simulink model "mpc_cvxgen"  (R2015b)
settings: Solver=VariableStepAuto  StartTime=0.0  StopTime=15  FixedStep=Ts  RelTol=1e-3
InitFcn:
  | mpc_trajectory_data_callback
values from neighbouring files (symbols this model uses):
  Ts = 0.1    [init_mpc_test.m]
undefined symbols (not defined in the file or in its folder): sCoeffs, sPolyorder, sTimes
undefined symbols (not defined in the file): CVXparameters
settings Model: Creator=Daniel  LastModifiedBy=mgreiff
settings SolverCC: AlgebraicLoopSolver=LineSearch

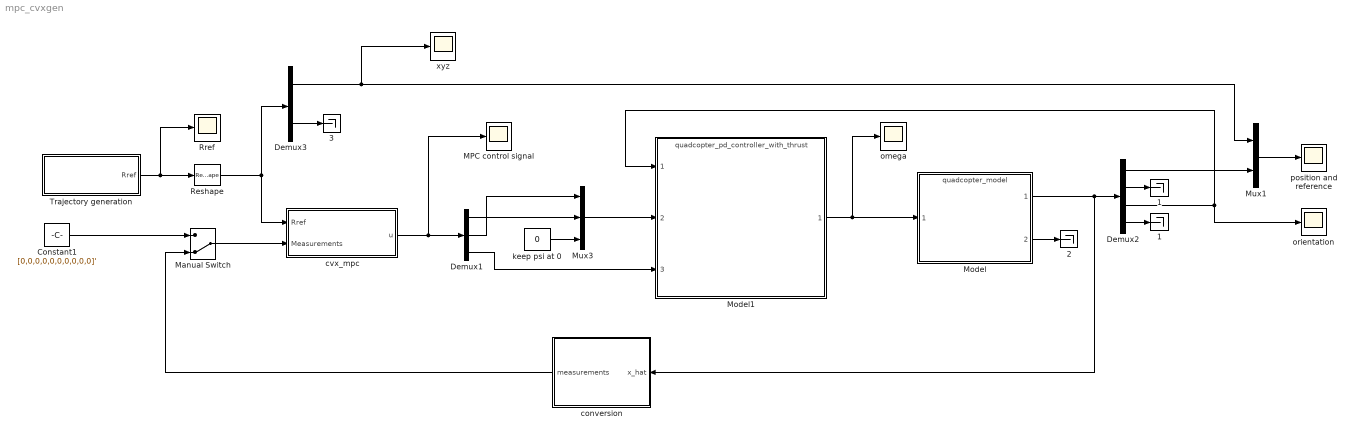
== system mpc_cvxgen ==
  "   1" : Terminator
  "   2" : Terminator
  "   3" : Terminator
  "  1" : Terminator
  Constant1 : Constant  Value=[0,0,0,0,0,0,0,0,0,0]'
  Demux1 : Demux  Outputs=3
  Demux2 : Demux  Outputs=[3,3,3,3]
  Demux3 : Demux  Outputs=[3,11*10-3]
  MPC control signal : Scope
  Manual Switch : ManualSwitch  CurrentSetting=0
  Model : ModelReference  ModelNameDialog=quadcopter_model.mdl  SimulationMode=Normal  ModelReferenceVersion=1.117  CopyOfModelName=quadcopter_model.mdl
  Model1 : ModelReference  ModelNameDialog=quadcopter_pd_controller_with_thrust.mdl  SimulationMode=Normal  ModelReferenceVersion=1.72  CopyOfModelName=quadcopter_pd_controller_with_thrust.mdl
  Mux1 : Mux  Inputs=2
  Mux3 : Mux  Inputs=3
  Reshape : Reshape
  Rref : Scope
  Trajectory generation : Subsystem
  conversion : Subsystem
  cvx_mpc : Subsystem  mask{md=CVXparameters}
      mask prompts: md "MPCData"
  keep psi at 0 : Constant  Value=0
  omega : Scope
  orientation : Scope
  position and reference : Scope
  xyz : Scope
  wires:
  Trajectory generation/1(Rref) -> Rref/1, Reshape/1
  cvx_mpc/1(u) -> MPC control signal/1, Demux1/1
  Demux1/3 -> Model1/3
  Mux3/1 -> Model1/2
  keep psi at 0/1 -> Mux3/3
  Demux1/2 -> Mux3/1
  Demux1/1 -> Mux3/2
  Demux2/2 -> "  1"/1
  Demux2/4 -> "   1"/1
  Demux2/3 -> Model1/1, orientation/1
  Model/1 -> Demux2/1, conversion/1(x_hat)
  Model/2 -> "   2"/1
  Model1/1 -> omega/1, Model/1
  Constant1/1 -> Manual Switch/1
  Manual Switch/1 -> cvx_mpc/2(Measurements)
  conversion/1(measurements) -> Manual Switch/2
  Reshape/1 -> Demux3/1, cvx_mpc/1(Rref)
  Demux3/2 -> "   3"/1
  Demux3/1 -> Mux1/1, xyz/1
  Demux2/1 -> Mux1/2
  Mux1/1 -> position and reference/1

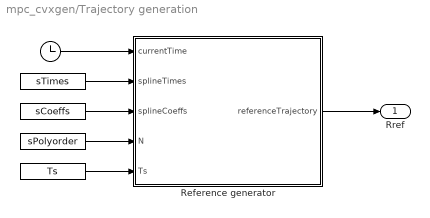
== system mpc_cvxgen/Trajectory generation ==
  " " : Constant  Value=Ts
  "  " : Constant  Value=sPolyorder
  "   " : Constant  Value=sCoeffs
  "    " : Constant  Value=sTimes
  "      " : Clock
  Reference generator : MATLAB Function  TreatAsAtomicUnit=on
  Rref : Outport
  wires:
  "      "/1 -> Reference generator/1(currentTime)
  "    "/1 -> Reference generator/2(splineTimes)
  "   "/1 -> Reference generator/3(splineCoeffs)
  "  "/1 -> Reference generator/4(N)
  " "/1 -> Reference generator/5(Ts)
  Reference generator/1(referenceTrajectory) -> Rref/1

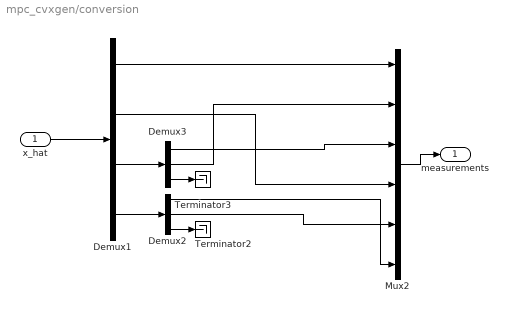
== system mpc_cvxgen/conversion ==
  x_hat : Inport
  Demux1 : Demux  Outputs=[3,3,3,3]
  Demux2 : Demux  Outputs=3
  Demux3 : Demux  Outputs=3
  Mux2 : Mux  Inputs=6
  Terminator2 : Terminator
  Terminator3 : Terminator
  measurements : Outport
  wires:
  Mux2/1 -> measurements/1
  x_hat/1 -> Demux1/1
  Demux1/1 -> Mux2/1
  Demux1/2 -> Mux2/4
  Demux2/3 -> Terminator2/1
  Demux1/4 -> Demux2/1
  Demux3/3 -> Terminator3/1
  Demux1/3 -> Demux3/1
  Demux3/2 -> Mux2/2
  Demux3/1 -> Mux2/3
  Demux2/1 -> Mux2/6
  Demux2/2 -> Mux2/5

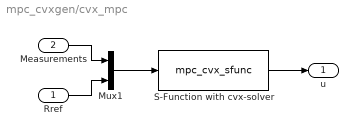
== system mpc_cvxgen/cvx_mpc ==
  Rref : Inport
  Measurements : Inport  Port=2
  Mux1 : Mux  Inputs=2
  S-Function with cvx-solver : S-Function  FunctionName=mpc_cvx_sfunc  Parameters=CVXparameters  SFunctionDeploymentMode=off  EnableBusSupport=off
  u : Outport
  wires:
  Measurements/1 -> Mux1/1
  Rref/1 -> Mux1/2
  S-Function with cvx-solver/1 -> u/1
  Mux1/1 -> S-Function with cvx-solver/1

== matlab function mpc_cvxgen/Trajectory generation/Reference generator ==
  data: currentTime input; referenceTrajectory output; splineTimes input; splineCoeffs input; N input; Ts input
function referenceTrajectory = fcn(currentTime, splineTimes, splineCoeffs, N, Ts)
%#codegen

predHorizon = 10 + 1; % Number of points on the prediction horizon

times = currentTime + Ts.* (0:predHorizon-1);
referenceTrajectory = zeros(10,predHorizon);

for ii = 1:predHorizon
    % Finds the spline to evaluate
    T = times(ii);
    splineNumber = sum(splineTimes <=  T);

    % Treats the case when the time is outside the defined interval [t_0,t_s]
    if splineNumber == 0
        %disp('Tried to evaluate spline before t_0, setting reference to the initial spline point.')
        T = splineTimes(1);
        splineNumber = 1;
    elseif T >= splineTimes(end)
        %disp('Tried to evaluate spline after t_s, keeping position in terinal spline point')
        T = splineTimes(end);
        splineNumber = length(splineCoeffs(:,1))/(N + 1);
    end
    % Evaluates splines and stores data in referenceTrajectory
    for dim = 1:3
        startIndex = (N + 1) * (splineNumber - 1) + 1;
        endIndex = (N + 1) * splineNumber;
        poscoeff = splineCoeffs(startIndex:endIndex,dim);
        poscoeff = poscoeff(end:-1:1); % Reverses for polyval
        tt = T - splineTimes(splineNumber);

        % Position
        referenceTrajectory(dim,ii) = polyval(poscoeff,tt);

        % Velocity
        poscoeff(end) = [];
        velcoeff = (length(poscoeff):-1:1)'.*poscoeff; 
        referenceTrajectory(dim + 3,ii) = polyval(velcoeff,tt);
    end
end
